simulink model "multirate_tests"  (R2019b)
settings: Solver=FixedStepDiscrete  StartTime=0  StopTime=20.0  RelTol=1e-3
libraries: dspsigops x18
settings Model: Creator=cyarp  LastModifiedBy=cyarp

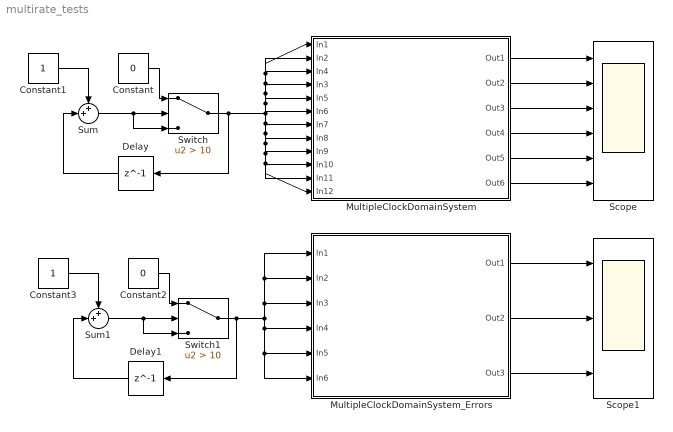
== system multirate_tests ==
  Constant : Constant  Value=0  OutDataTypeStr=single
  Constant1 : Constant  OutDataTypeStr=single
  Constant2 : Constant  Value=0  OutDataTypeStr=single
  Constant3 : Constant  OutDataTypeStr=single
  Delay : Delay  DelayLength=1  SampleTime=4
  Delay1 : Delay  DelayLength=1  SampleTime=4
  MultipleClockDomainSystem : Subsystem
  MultipleClockDomainSystem_Errors : Subsystem
  Scope : Scope  NumInputPorts=6
  Scope1 : Scope  NumInputPorts=3
  Sum : Sum  Inputs=++|
  Sum1 : Sum  Inputs=++|
  Switch : Switch  Criteria=u2 > Threshold  Threshold=10
  Switch1 : Switch  Criteria=u2 > Threshold  Threshold=10
  wires:
  MultipleClockDomainSystem/1(Out1) -> Scope/1
  MultipleClockDomainSystem/2(Out2) -> Scope/2
  MultipleClockDomainSystem/3(Out3) -> Scope/3
  MultipleClockDomainSystem/4(Out4) -> Scope/4
  MultipleClockDomainSystem/5(Out5) -> Scope/5
  Delay/1 -> Sum/2
  Switch/1 -> Delay/1, MultipleClockDomainSystem/1(In1), MultipleClockDomainSystem/2(In2), MultipleClockDomainSystem/3(In4), MultipleClockDomainSystem/4(In3), MultipleClockDomainSystem/5(In5), MultipleClockDomainSystem/12(In12), MultipleClockDomainSystem/11(In11), MultipleClockDomainSystem/10(In10), MultipleClockDomainSystem/9(In9), MultipleClockDomainSystem/8(In8), MultipleClockDomainSystem/7(In7), MultipleClockDomainSystem/6(In6)
  Sum/1 -> Switch/2, Switch/3
  Constant/1 -> Switch/1
  Constant1/1 -> Sum/1
  MultipleClockDomainSystem/6(Out6) -> Scope/6
  Constant2/1 -> Switch1/1
  Delay1/1 -> Sum1/2
  Constant3/1 -> Sum1/1
  Switch1/1 -> MultipleClockDomainSystem_Errors/6(In6), MultipleClockDomainSystem_Errors/5(In5), MultipleClockDomainSystem_Errors/4(In4), MultipleClockDomainSystem_Errors/3(In3), MultipleClockDomainSystem_Errors/2(In2), MultipleClockDomainSystem_Errors/1(In1), Delay1/1
  Sum1/1 -> Switch1/2, Switch1/3
  MultipleClockDomainSystem_Errors/1(Out1) -> Scope1/1
  MultipleClockDomainSystem_Errors/2(Out2) -> Scope1/2
  MultipleClockDomainSystem_Errors/3(Out3) -> Scope1/3

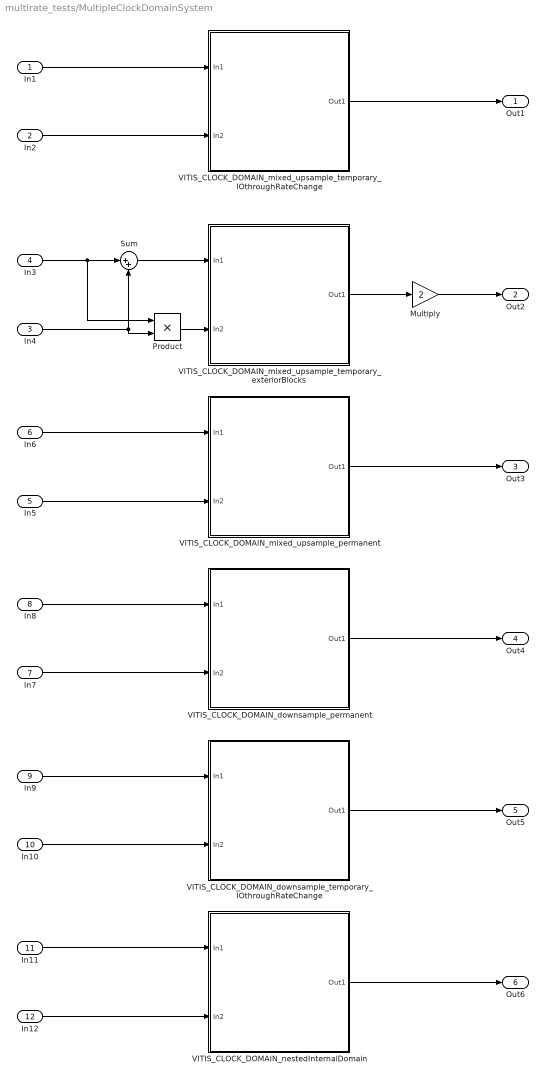
== system multirate_tests/MultipleClockDomainSystem ==
  In1 : Inport
  In2 : Inport  Port=2
  In4 : Inport  Port=3
  In3 : Inport  Port=4
  In5 : Inport  Port=5
  In6 : Inport  Port=6
  In7 : Inport  Port=7
  In8 : Inport  Port=8
  In9 : Inport  Port=9
  In10 : Inport  Port=10
  In11 : Inport  Port=11
  In12 : Inport  Port=12
  Multiply : Gain  Gain=2
  Product : Product
  Sum : Sum  Inputs=|++
  VITIS_CLOCK_DOMAIN_downsample_permanent : Subsystem
  VITIS_CLOCK_DOMAIN_downsample_temporary_IOthroughRateChange : Subsystem
  VITIS_CLOCK_DOMAIN_mixed_upsample_permanent : Subsystem
  VITIS_CLOCK_DOMAIN_mixed_upsample_temporary_IOthroughRateChange : Subsystem
  VITIS_CLOCK_DOMAIN_mixed_upsample_temporary_exteriorBlocks : Subsystem
  VITIS_CLOCK_DOMAIN_nestedInternalDomain : Subsystem
  Out1 : Outport
  Out2 : Outport  Port=2
  Out3 : Outport  Port=3
  Out4 : Outport  Port=4
  Out5 : Outport  Port=5
  Out6 : Outport  Port=6
  wires:
  In1/1 -> VITIS_CLOCK_DOMAIN_mixed_upsample_temporary_IOthroughRateChange/1(In1)
  In2/1 -> VITIS_CLOCK_DOMAIN_mixed_upsample_temporary_IOthroughRateChange/2(In2)
  VITIS_CLOCK_DOMAIN_mixed_upsample_temporary_IOthroughRateChange/1(Out1) -> Out1/1
  In4/1 -> Sum/2, Product/2
  In3/1 -> Product/1, Sum/1
  Sum/1 -> VITIS_CLOCK_DOMAIN_mixed_upsample_temporary_exteriorBlocks/1(In1)
  Product/1 -> VITIS_CLOCK_DOMAIN_mixed_upsample_temporary_exteriorBlocks/2(In2)
  VITIS_CLOCK_DOMAIN_mixed_upsample_temporary_exteriorBlocks/1(Out1) -> Multiply/1
  Multiply/1 -> Out2/1
  VITIS_CLOCK_DOMAIN_mixed_upsample_permanent/1(Out1) -> Out3/1
  In6/1 -> VITIS_CLOCK_DOMAIN_mixed_upsample_permanent/1(In1)
  In5/1 -> VITIS_CLOCK_DOMAIN_mixed_upsample_permanent/2(In2)
  In8/1 -> VITIS_CLOCK_DOMAIN_downsample_permanent/1(In1)
  VITIS_CLOCK_DOMAIN_downsample_permanent/1(Out1) -> Out4/1
  In7/1 -> VITIS_CLOCK_DOMAIN_downsample_permanent/2(In2)
  In9/1 -> VITIS_CLOCK_DOMAIN_downsample_temporary_IOthroughRateChange/1(In1)
  In10/1 -> VITIS_CLOCK_DOMAIN_downsample_temporary_IOthroughRateChange/2(In2)
  VITIS_CLOCK_DOMAIN_downsample_temporary_IOthroughRateChange/1(Out1) -> Out5/1
  In11/1 -> VITIS_CLOCK_DOMAIN_nestedInternalDomain/1(In1)
  In12/1 -> VITIS_CLOCK_DOMAIN_nestedInternalDomain/2(In2)
  VITIS_CLOCK_DOMAIN_nestedInternalDomain/1(Out1) -> Out6/1

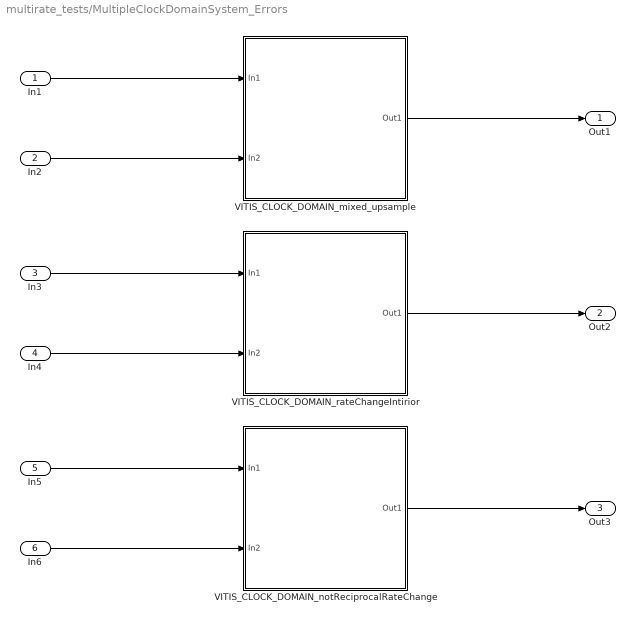
== system multirate_tests/MultipleClockDomainSystem_Errors ==
  In1 : Inport
  In2 : Inport  Port=2
  In3 : Inport  Port=3
  In4 : Inport  Port=4
  In5 : Inport  Port=5
  In6 : Inport  Port=6
  VITIS_CLOCK_DOMAIN_mixed_upsample : Subsystem
  VITIS_CLOCK_DOMAIN_notReciprocalRateChange : Subsystem
  VITIS_CLOCK_DOMAIN_rateChangeIntirior : Subsystem
  Out1 : Outport
  Out2 : Outport  Port=2
  Out3 : Outport  Port=3
  wires:
  In1/1 -> VITIS_CLOCK_DOMAIN_mixed_upsample/1(In1)
  In2/1 -> VITIS_CLOCK_DOMAIN_mixed_upsample/2(In2)
  VITIS_CLOCK_DOMAIN_mixed_upsample/1(Out1) -> Out1/1
  In4/1 -> VITIS_CLOCK_DOMAIN_rateChangeIntirior/2(In2)
  In3/1 -> VITIS_CLOCK_DOMAIN_rateChangeIntirior/1(In1)
  In6/1 -> VITIS_CLOCK_DOMAIN_notReciprocalRateChange/2(In2)
  In5/1 -> VITIS_CLOCK_DOMAIN_notReciprocalRateChange/1(In1)
  VITIS_CLOCK_DOMAIN_rateChangeIntirior/1(Out1) -> Out2/1
  VITIS_CLOCK_DOMAIN_notReciprocalRateChange/1(Out1) -> Out3/1

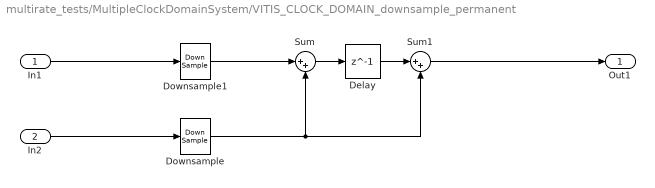
== system multirate_tests/MultipleClockDomainSystem/VITIS_CLOCK_DOMAIN_downsample_permanent ==
  In1 : Inport
  In2 : Inport  Port=2
  Delay : Delay  DelayLength=1
  Downsample : DownSample  RateOptions=Allow multirate processing
  Downsample1 : DownSample  RateOptions=Allow multirate processing
  Sum : Sum  Inputs=|++
  Sum1 : Sum  Inputs=|++
  Out1 : Outport
  wires:
  Sum1/1 -> Out1/1
  Sum/1 -> Delay/1
  Downsample/1 -> Sum1/2, Sum/2
  Delay/1 -> Sum1/1
  In1/1 -> Downsample1/1
  In2/1 -> Downsample/1
  Downsample1/1 -> Sum/1

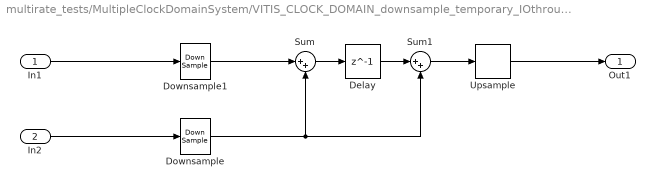
== system multirate_tests/MultipleClockDomainSystem/VITIS_CLOCK_DOMAIN_downsample_temporary_IOthroughRateChange ==
  In1 : Inport
  In2 : Inport  Port=2
  Delay : Delay  DelayLength=1
  Downsample : DownSample  N=4  RateOptions=Allow multirate processing
  Downsample1 : DownSample  N=4  RateOptions=Allow multirate processing
  Sum : Sum  Inputs=|++
  Sum1 : Sum  Inputs=|++
  Upsample : dspsigops/Upsample  N=4  phase=0  RateOptions=Allow multirate processing  ic=0  mode=Unused parameter value
  Out1 : Outport
  wires:
  Upsample/1 -> Out1/1
  Sum1/1 -> Upsample/1
  Sum/1 -> Delay/1
  Downsample/1 -> Sum1/2, Sum/2
  Delay/1 -> Sum1/1
  In1/1 -> Downsample1/1
  In2/1 -> Downsample/1
  Downsample1/1 -> Sum/1

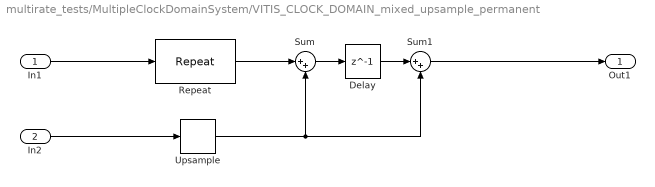
== system multirate_tests/MultipleClockDomainSystem/VITIS_CLOCK_DOMAIN_mixed_upsample_permanent ==
  In1 : Inport
  In2 : Inport  Port=2
  Delay : Delay  DelayLength=1
  Repeat : dspsigops/Repeat  N=4  InputProcessing=Columns as channels (frame based)  RateOptions=Allow multirate processing  ic=0  mode=Unused parameter value
      settings: SourceProductName=DSP System Toolbox
  Sum : Sum  Inputs=|++
  Sum1 : Sum  Inputs=|++
  Upsample : dspsigops/Upsample  N=4  phase=0  RateOptions=Allow multirate processing  ic=0  mode=Unused parameter value
  Out1 : Outport
  wires:
  Sum1/1 -> Out1/1
  Sum/1 -> Delay/1
  Upsample/1 -> Sum1/2, Sum/2
  Delay/1 -> Sum1/1
  In1/1 -> Repeat/1
  In2/1 -> Upsample/1
  Repeat/1 -> Sum/1

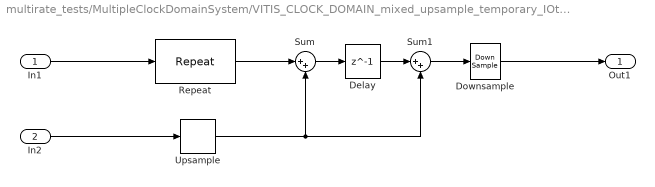
== system multirate_tests/MultipleClockDomainSystem/VITIS_CLOCK_DOMAIN_mixed_upsample_temporary_IOthroughRateChange ==
  In1 : Inport
  In2 : Inport  Port=2
  Delay : Delay  DelayLength=1
  Downsample : DownSample  N=4  RateOptions=Allow multirate processing
  Repeat : dspsigops/Repeat  N=4  InputProcessing=Columns as channels (frame based)  RateOptions=Allow multirate processing  ic=0  mode=Unused parameter value
      settings: SourceProductName=DSP System Toolbox
  Sum : Sum  Inputs=|++
  Sum1 : Sum  Inputs=|++
  Upsample : dspsigops/Upsample  N=4  phase=0  RateOptions=Allow multirate processing  ic=0  mode=Unused parameter value
  Out1 : Outport
  wires:
  Downsample/1 -> Out1/1
  Sum1/1 -> Downsample/1
  Sum/1 -> Delay/1
  Upsample/1 -> Sum1/2, Sum/2
  Delay/1 -> Sum1/1
  In1/1 -> Repeat/1
  In2/1 -> Upsample/1
  Repeat/1 -> Sum/1

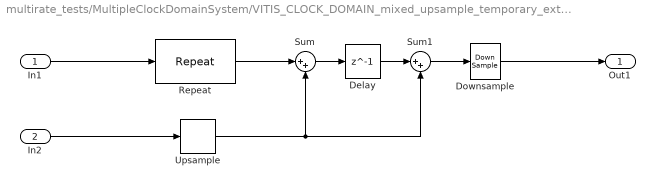
== system multirate_tests/MultipleClockDomainSystem/VITIS_CLOCK_DOMAIN_mixed_upsample_temporary_exteriorBlocks ==
  In1 : Inport
  In2 : Inport  Port=2
  Delay : Delay  DelayLength=1
  Downsample : DownSample  N=4  RateOptions=Allow multirate processing
  Repeat : dspsigops/Repeat  N=4  InputProcessing=Columns as channels (frame based)  RateOptions=Allow multirate processing  ic=0  mode=Unused parameter value
      settings: SourceProductName=DSP System Toolbox
  Sum : Sum  Inputs=|++
  Sum1 : Sum  Inputs=|++
  Upsample : dspsigops/Upsample  N=4  phase=0  RateOptions=Allow multirate processing  ic=0  mode=Unused parameter value
  Out1 : Outport
  wires:
  Downsample/1 -> Out1/1
  Sum1/1 -> Downsample/1
  Sum/1 -> Delay/1
  Upsample/1 -> Sum1/2, Sum/2
  Delay/1 -> Sum1/1
  In1/1 -> Repeat/1
  In2/1 -> Upsample/1
  Repeat/1 -> Sum/1

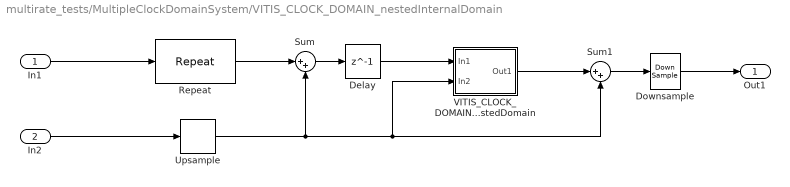
== system multirate_tests/MultipleClockDomainSystem/VITIS_CLOCK_DOMAIN_nestedInternalDomain ==
  In1 : Inport
  In2 : Inport  Port=2
  Delay : Delay  DelayLength=1
  Downsample : DownSample  N=4  RateOptions=Allow multirate processing
  Repeat : dspsigops/Repeat  N=4  InputProcessing=Columns as channels (frame based)  RateOptions=Allow multirate processing  ic=0  mode=Unused parameter value
      settings: SourceProductName=DSP System Toolbox
  Sum : Sum  Inputs=|++
  Sum1 : Sum  Inputs=|++
  Upsample : dspsigops/Upsample  N=4  phase=0  RateOptions=Allow multirate processing  ic=0  mode=Unused parameter value
  VITIS_CLOCK_DOMAIN_nestedDomain : Subsystem
  Out1 : Outport
  wires:
  Downsample/1 -> Out1/1
  Sum1/1 -> Downsample/1
  Sum/1 -> Delay/1
  Upsample/1 -> VITIS_CLOCK_DOMAIN_nestedDomain/2(In2), Sum1/2, Sum/2
  In1/1 -> Repeat/1
  In2/1 -> Upsample/1
  Repeat/1 -> Sum/1
  Delay/1 -> VITIS_CLOCK_DOMAIN_nestedDomain/1(In1)
  VITIS_CLOCK_DOMAIN_nestedDomain/1(Out1) -> Sum1/1

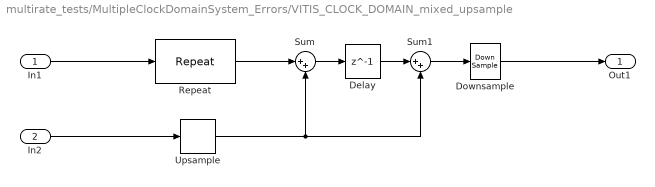
== system multirate_tests/MultipleClockDomainSystem_Errors/VITIS_CLOCK_DOMAIN_mixed_upsample ==
  In1 : Inport
  In2 : Inport  Port=2
  Delay : Delay  DelayLength=1
  Downsample : DownSample  N=4  RateOptions=Allow multirate processing
  Repeat : dspsigops/Repeat  N=4  InputProcessing=Columns as channels (frame based)  RateOptions=Allow multirate processing  ic=0  mode=Unused parameter value
      settings: SourceProductName=DSP System Toolbox
  Sum : Sum  Inputs=|++
  Sum1 : Sum  Inputs=|++
  Upsample : dspsigops/Upsample  N=8  phase=0  RateOptions=Allow multirate processing  ic=0  mode=Unused parameter value
  Out1 : Outport
  wires:
  Downsample/1 -> Out1/1
  Sum1/1 -> Downsample/1
  Sum/1 -> Delay/1
  Upsample/1 -> Sum1/2, Sum/2
  Delay/1 -> Sum1/1
  In1/1 -> Repeat/1
  In2/1 -> Upsample/1
  Repeat/1 -> Sum/1

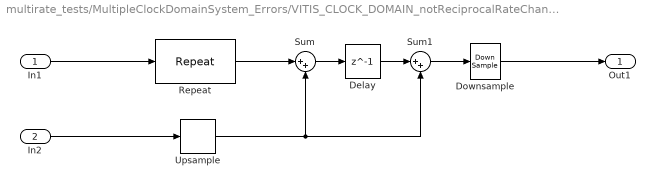
== system multirate_tests/MultipleClockDomainSystem_Errors/VITIS_CLOCK_DOMAIN_notReciprocalRateChange ==
  In1 : Inport
  In2 : Inport  Port=2
  Delay : Delay  DelayLength=1
  Downsample : DownSample  RateOptions=Allow multirate processing
  Repeat : dspsigops/Repeat  N=4  InputProcessing=Columns as channels (frame based)  RateOptions=Allow multirate processing  ic=0  mode=Unused parameter value
      settings: SourceProductName=DSP System Toolbox
  Sum : Sum  Inputs=|++
  Sum1 : Sum  Inputs=|++
  Upsample : dspsigops/Upsample  N=4  phase=0  RateOptions=Allow multirate processing  ic=0  mode=Unused parameter value
  Out1 : Outport
  wires:
  Downsample/1 -> Out1/1
  Sum1/1 -> Downsample/1
  Sum/1 -> Delay/1
  Upsample/1 -> Sum1/2, Sum/2
  Delay/1 -> Sum1/1
  In1/1 -> Repeat/1
  In2/1 -> Upsample/1
  Repeat/1 -> Sum/1

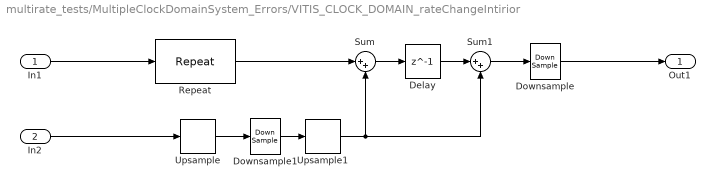
== system multirate_tests/MultipleClockDomainSystem_Errors/VITIS_CLOCK_DOMAIN_rateChangeIntirior ==
  In1 : Inport
  In2 : Inport  Port=2
  Delay : Delay  DelayLength=1
  Downsample : DownSample  N=4  RateOptions=Allow multirate processing
  Downsample1 : DownSample  RateOptions=Allow multirate processing
  Repeat : dspsigops/Repeat  N=4  InputProcessing=Columns as channels (frame based)  RateOptions=Allow multirate processing  ic=0  mode=Unused parameter value
      settings: SourceProductName=DSP System Toolbox
  Sum : Sum  Inputs=|++
  Sum1 : Sum  Inputs=|++
  Upsample : dspsigops/Upsample  N=4  phase=0  RateOptions=Allow multirate processing  ic=0  mode=Unused parameter value
  Upsample1 : dspsigops/Upsample  N=2  phase=0  RateOptions=Allow multirate processing  ic=0  mode=Unused parameter value
  Out1 : Outport
  wires:
  Downsample/1 -> Out1/1
  Sum1/1 -> Downsample/1
  Sum/1 -> Delay/1
  Upsample/1 -> Downsample1/1
  Delay/1 -> Sum1/1
  In1/1 -> Repeat/1
  In2/1 -> Upsample/1
  Repeat/1 -> Sum/1
  Downsample1/1 -> Upsample1/1
  Upsample1/1 -> Sum1/2, Sum/2

== system multirate_tests/MultipleClockDomainSystem/VITIS_CLOCK_DOMAIN_nestedInternalDomain/VITIS_CLOCK_DOMAIN_nestedDomain ==
  In1 : Inport
  In2 : Inport  Port=2
  Delay1 : Delay  DelayLength=1
  Downsample1 : DownSample  RateOptions=Allow multirate processing
  Sum2 : Sum  Inputs=|++
  Upsample1 : dspsigops/Upsample  N=2  phase=0  RateOptions=Allow multirate processing  ic=0  mode=Unused parameter value
  Upsample2 : dspsigops/Upsample  N=2  phase=0  RateOptions=Allow multirate processing  ic=0  mode=Unused parameter value
  Out1 : Outport
  wires:
  Downsample1/1 -> Out1/1
  In2/1 -> Upsample2/1
  In1/1 -> Upsample1/1
  Upsample2/1 -> Delay1/1
  Upsample1/1 -> Sum2/1
  Delay1/1 -> Sum2/2
  Sum2/1 -> Downsample1/1
